simulink model "ZEM_Example"  (R2020b)
settings: Solver=ode4  StartTime=0.0  StopTime=simTime  FixedStep=h  RelTol=1e-3
values from neighbouring files (symbols this model uses):
  Beta = 0    [ZeroEffortMiss.m]
  N_prime = 4    [ZeroEffortMiss.m]
  nt = 3    [ZeroEffortMiss.m]
  Rm1 = 0    [ZeroEffortMiss.m]
  Rm2 = 10000    [ZeroEffortMiss.m]
  Rt1 = 40000    [ZeroEffortMiss.m]
  Rt2 = Rm2    (= 10000)    [ZeroEffortMiss.m]
  Tf = simTime    (= 10)    [ZeroEffortMiss.m]
  Vm1_0 = Vm*cos(L+HE+Lambda)    [ZeroEffortMiss.m]
  Vm2_0 = Vm*sin(L+HE+Lambda)    [ZeroEffortMiss.m]
  Vt = 1000    [ZeroEffortMiss.m]
  Vt1_0 = -Vt*cos(Beta)    [ZeroEffortMiss.m]
  Vt2_0 = Vt*sin(Beta)    [ZeroEffortMiss.m]
libraries: simulink x1
settings Model: Creator=dariusmensah  LastModifiedBy=dariusmensah

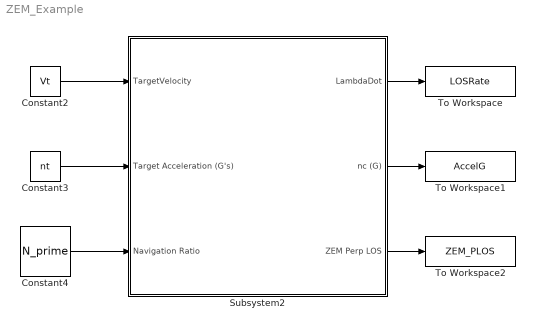
== system ZEM_Example ==
  Constant2 : Constant  Value=Vt
  Constant3 : Constant  Value=nt
  Constant4 : Constant  Value=N_prime
  Subsystem2 : Subsystem
  To Workspace : ToWorkspace  VariableName=LOSRate  SaveFormat=Structure With Time  SampleTime=-1
  To Workspace1 : ToWorkspace  VariableName=AccelG  SaveFormat=Structure With Time  SampleTime=-1
  To Workspace2 : ToWorkspace  VariableName=ZEM_PLOS  SaveFormat=Structure With Time  SampleTime=-1
  wires:
  Constant2/1 -> Subsystem2/1(TargetVelocity)
  Constant4/1 -> Subsystem2/3(Navigation Ratio)
  Constant3/1 -> Subsystem2/2(Target Acceleration (G's))
  Subsystem2/3(ZEM Perp LOS) -> To Workspace2/1
  Subsystem2/2(nc (G)) -> To Workspace1/1
  Subsystem2/1(LambdaDot) -> To Workspace/1

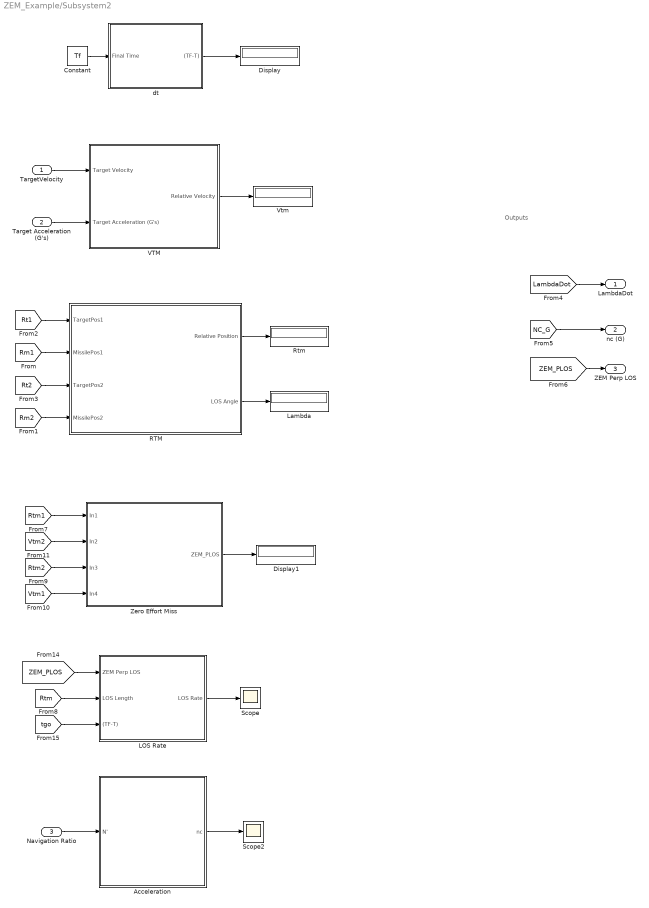
== system ZEM_Example/Subsystem2 ==
  note: Outputs
  TargetVelocity : Inport
  Target Acceleration (G's) : Inport  Port=2
  Navigation Ratio : Inport  Port=3
  Acceleration : Subsystem
  Constant : Constant  Value=Tf
  Display : Display
  Display1 : Display
  LOS Rate : Subsystem
  Lambda : Display
  RTM : Subsystem
  Rtm : Display
  Scope : Scope
  Scope2 : Scope
  VTM : Subsystem
  Vtm : Display
  Zero Effort Miss : Subsystem
  dt : Subsystem
  LambdaDot : Outport
  nc (G) : Outport  Port=2
  ZEM Perp LOS : Outport  Port=3
  wires:
  TargetVelocity/1 -> VTM/1(Target Velocity)
  [Rm2] -> RTM/4(MissilePos2)
  [Rt1] -> RTM/1(TargetPos1)
  VTM/1(Relative Velocity) -> Vtm/1
  RTM/1(Relative Position) -> Rtm/1
  [Rt2] -> RTM/3(TargetPos2)
  [Rm1] -> RTM/2(MissilePos1)
  Target Acceleration (G's)/1 -> VTM/2(Target Acceleration (G's))
  RTM/2(LOS Angle) -> Lambda/1
  Navigation Ratio/1 -> Acceleration/1(N')
  Acceleration/1(nc) -> Scope2/1
  [ZEM_PLOS] -> LOS Rate/1(ZEM Perp LOS)
  [Rtm] -> LOS Rate/2(LOS Length)
  [tgo] -> LOS Rate/3((TF-T))
  LOS Rate/1(LOS Rate) -> Scope/1
  Constant/1 -> dt/1(Final Time)
  dt/1((TF-T)) -> Display/1
  Zero Effort Miss/1(ZEM_PLOS) -> Display1/1
  [LambdaDot] -> LambdaDot/1
  [NC_G] -> nc (G)/1
  [ZEM_PLOS] -> ZEM Perp LOS/1
  [Rtm1] -> Zero Effort Miss/1(In1)
  [Vtm2] -> Zero Effort Miss/2(In2)
  [Rtm2] -> Zero Effort Miss/3(In3)
  [Vtm1] -> Zero Effort Miss/4(In4)

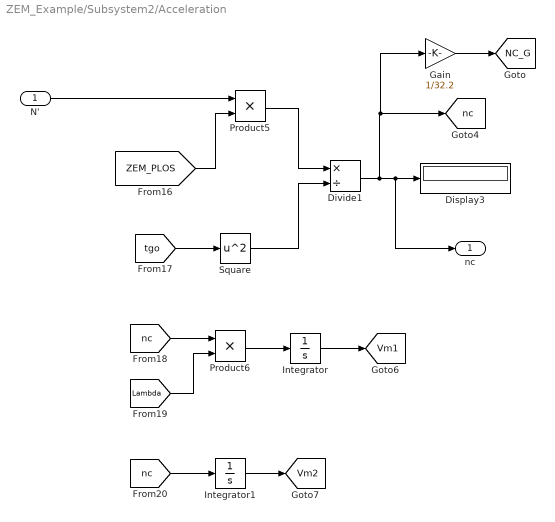
== system ZEM_Example/Subsystem2/Acceleration ==
  N' : Inport
  Display3 : Display
  Divide1 : Product  Inputs=*/
  Gain : Gain  Gain=1/32.2
  Integrator : Integrator  InitialCondition=Vm1_0
  Integrator1 : Integrator  InitialCondition=Vm2_0
  Product5 : Product
  Product6 : Product
  Square : Math  Operator=square  SaturateOnIntegerOverflow=on
  nc : Outport
  tag scope: NC_G=global, Vm1=global, Vm2=global, nc=global
  wires:
  [nc] -> Product6/1
  [tgo] -> Square/1
  N'/1 -> Product5/1
  Integrator1/1 -> [Vm2]
  [Lambda] -> Product6/2
  Integrator/1 -> [Vm1]
  Square/1 -> Divide1/2
  Product5/1 -> Divide1/1
  [ZEM_PLOS] -> Product5/2
  Divide1/1 -> Gain/1, [nc], nc/1, Display3/1
  Product6/1 -> Integrator/1
  Gain/1 -> [NC_G]
  [nc] -> Integrator1/1

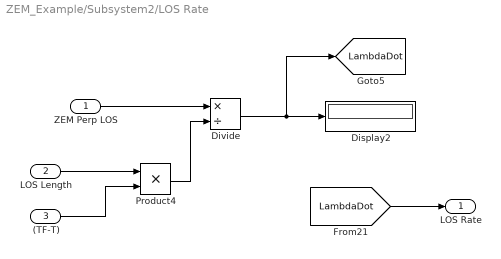
== system ZEM_Example/Subsystem2/LOS Rate ==
  ZEM Perp LOS : Inport
  LOS Length : Inport  Port=2
  (TF-T) : Inport  Port=3
  Display2 : Display
  Divide : Product  Inputs=*/
  Product4 : Product
  LOS Rate : Outport
  tag scope: LambdaDot=global
  wires:
  (TF-T)/1 -> Product4/2
  LOS Length/1 -> Product4/1
  Divide/1 -> [LambdaDot], Display2/1
  [LambdaDot] -> LOS Rate/1
  Product4/1 -> Divide/2
  ZEM Perp LOS/1 -> Divide/1

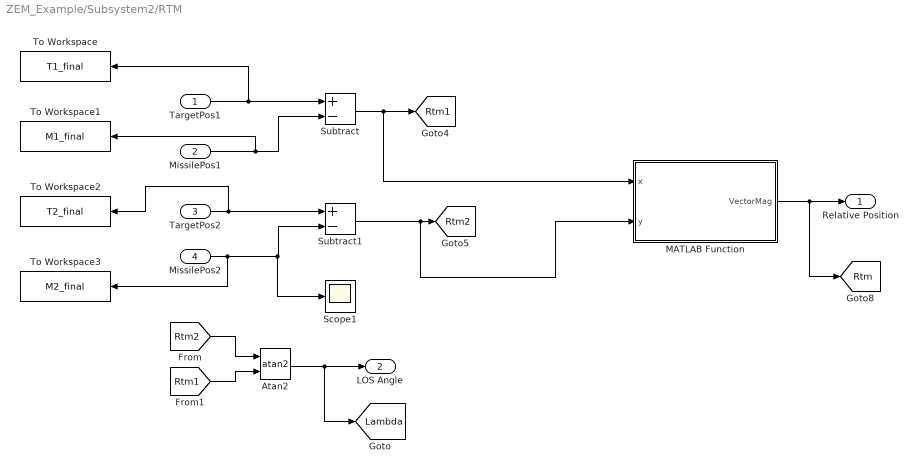
== system ZEM_Example/Subsystem2/RTM ==
  TargetPos1 : Inport
  MissilePos1 : Inport  Port=2
  TargetPos2 : Inport  Port=3
  MissilePos2 : Inport  Port=4
  Atan2 : Trigonometry  Operator=atan2
  MATLAB Function : MATLAB Function  TreatAsAtomicUnit=on
  Scope1 : Scope
  Subtract : Sum  Inputs=+-
  Subtract1 : Sum  Inputs=+-
  To Workspace : ToWorkspace  VariableName=T1_final  SaveFormat=Structure With Time  SampleTime=-1
  To Workspace1 : ToWorkspace  VariableName=M1_final  SaveFormat=Structure With Time  SampleTime=-1
  To Workspace2 : ToWorkspace  VariableName=T2_final  SaveFormat=Structure With Time  SampleTime=-1
  To Workspace3 : ToWorkspace  VariableName=M2_final  SaveFormat=Structure With Time  SampleTime=-1
  Relative Position : Outport
  LOS Angle : Outport  Port=2
  tag scope: Lambda=global, Rtm1=global, Rtm2=global, Rtm=global
  wires:
  MissilePos2/1 -> To Workspace3/1, Scope1/1, Subtract1/2
  Subtract1/1 -> MATLAB Function/2(y), [Rtm2]
  TargetPos1/1 -> To Workspace/1, Subtract/1
  TargetPos2/1 -> To Workspace2/1, Subtract1/1
  Subtract/1 -> MATLAB Function/1(x), [Rtm1]
  MissilePos1/1 -> To Workspace1/1, Subtract/2
  [Rtm1] -> Atan2/2
  [Rtm2] -> Atan2/1
  Atan2/1 -> [Lambda], LOS Angle/1
  MATLAB Function/1(VectorMag) -> [Rtm], Relative Position/1

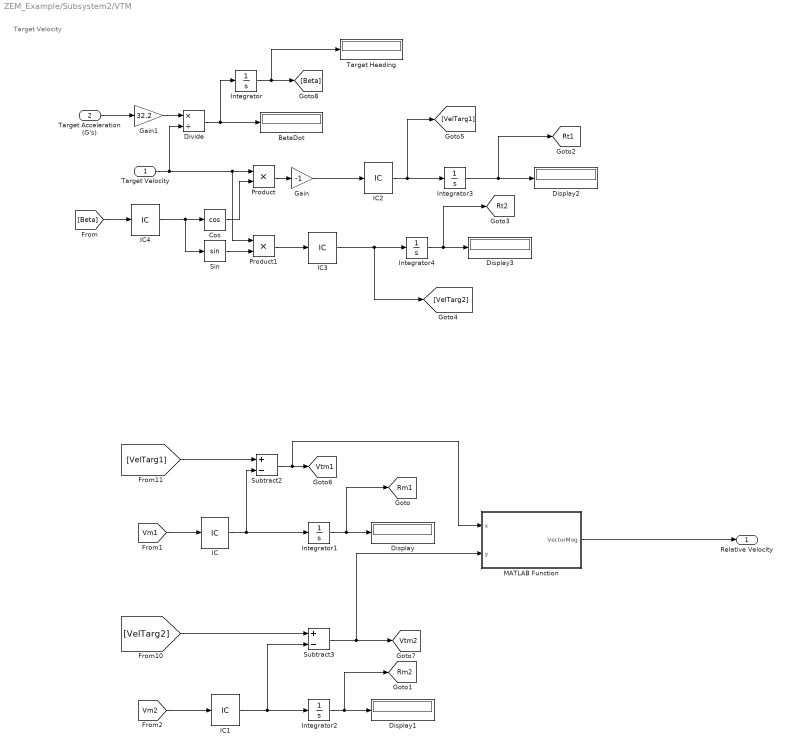
== system ZEM_Example/Subsystem2/VTM ==
  note: Target Velocity
  Target Velocity : Inport
  Target Acceleration (G's) : Inport  Port=2
  BetaDot : Display
  Cos : Trigonometry  Operator=cos
  Display{,1..3} (4 alike) : Display
  Divide : Product  Inputs=*/
  Gain : Gain  Gain=-1
  Gain1 : Gain  Gain=32.2
  IC : InitialCondition  Value=Vm1_0
  IC1 : InitialCondition  Value=Vm2_0
  IC2 : InitialCondition  Value=Vt1_0
  IC3 : InitialCondition  Value=Vt2_0
  IC4 : InitialCondition  Value=Beta
  Integrator : Integrator
  Integrator1 : Integrator  InitialCondition=Rm1
  Integrator2 : Integrator  InitialCondition=Rm2
  Integrator3 : Integrator  InitialCondition=Rt1
  Integrator4 : Integrator  InitialCondition=Rt2
  MATLAB Function : MATLAB Function  TreatAsAtomicUnit=on
  Product : Product
  Product1 : Product
  Sin : Trigonometry
  Subtract2 : Sum  Inputs=+-
  Subtract3 : Sum  Inputs=+-
  Target Heading : Display
  Relative Velocity : Outport
  tag scope: Rm1=global, Rm2=global, Rt1=global, Rt2=global, Vtm1=global, Vtm2=global
  wires:
  MATLAB Function/1(VectorMag) -> Relative Velocity/1
  [Vm1] -> IC/1
  Sin/1 -> Product1/2
  [VelTarg1] -> Subtract2/1
  Product/1 -> Gain/1
  Target Velocity/1 -> Divide/2, Product1/1, Product/1
  Subtract2/1 -> MATLAB Function/1(x), [Vtm1]
  [VelTarg2] -> Subtract3/1
  Cos/1 -> Product/2
  Product1/1 -> IC3/1
  Subtract3/1 -> MATLAB Function/2(y), [Vtm2]
  Integrator4/1 -> [Rt2], Display3/1
  IC/1 -> Integrator1/1, Subtract2/2
  [Vm2] -> IC1/1
  [Beta] -> IC4/1
  IC2/1 -> [VelTarg1], Integrator3/1
  Integrator2/1 -> [Rm2], Display1/1
  IC3/1 -> [VelTarg2], Integrator4/1
  Integrator1/1 -> Display/1, [Rm1]
  Integrator3/1 -> Display2/1, [Rt1]
  IC1/1 -> Subtract3/2, Integrator2/1
  Gain/1 -> IC2/1
  Divide/1 -> BetaDot/1, Integrator/1
  IC4/1 -> Sin/1, Cos/1
  Integrator/1 -> Target Heading/1, [Beta]
  Target Acceleration (G's)/1 -> Gain1/1
  Gain1/1 -> Divide/1

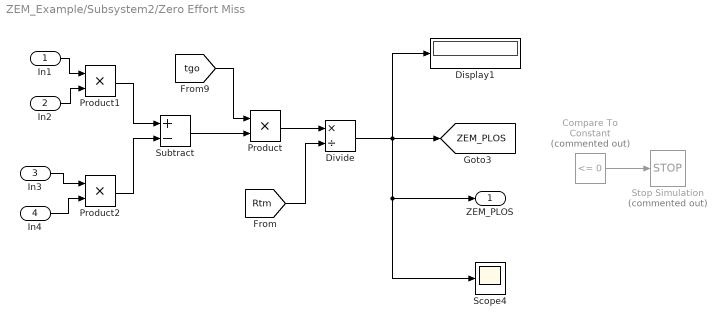
== system ZEM_Example/Subsystem2/Zero Effort Miss ==
  In1 : Inport
  In2 : Inport  Port=2
  In3 : Inport  Port=3
  In4 : Inport  Port=4
  Compare To Constant : simulink/Logic and Bit Operations/Compare To Constant  Commented=on  relop=<=  const=0  OutDataTypeStr=boolean
  Display1 : Display
  Divide : Product  Inputs=*/
  Product : Product
  Product1 : Product
  Product2 : Product
  Scope4 : Scope
  Stop Simulation : Stop  Commented=on
  Subtract : Sum  Inputs=+-
  ZEM_PLOS : Outport
  tag scope: ZEM_PLOS=global
  wires:
  Compare To Constant/1 -> Stop Simulation/1
  In2/1 -> Product1/2
  In1/1 -> Product1/1
  Product1/1 -> Subtract/1
  In3/1 -> Product2/1
  In4/1 -> Product2/2
  Product2/1 -> Subtract/2
  Subtract/1 -> Product/2
  [tgo] -> Product/1
  Product/1 -> Divide/1
  [Rtm] -> Divide/2
  Divide/1 -> Display1/1, Scope4/1, ZEM_PLOS/1, [ZEM_PLOS]

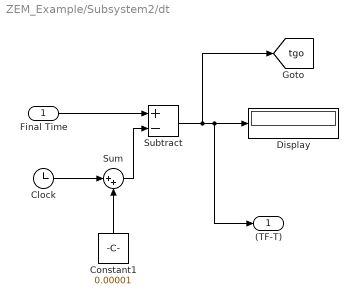
== system ZEM_Example/Subsystem2/dt ==
  Final Time : Inport
  Clock : Clock
  Constant1 : Constant  Value=0.00001
  Display : Display
  Subtract : Sum  Inputs=+-
  Sum : Sum  Inputs=|++
  (TF-T) : Outport
  tag scope: tgo=global
  wires:
  Final Time/1 -> Subtract/1
  Sum/1 -> Subtract/2
  Clock/1 -> Sum/1
  Subtract/1 -> [tgo], (TF-T)/1, Display/1
  Constant1/1 -> Sum/2

== matlab function ZEM_Example/Subsystem2/RTM/MATLAB Function ==
  data: x input; VectorMag output; y input
function VectorMag = fcn(x,y)

a = x^2 + y^2;
VectorMag = sqrt(a);
end

== matlab function ZEM_Example/Subsystem2/VTM/MATLAB Function ==
  data: x input; VectorMag output; y input
function VectorMag = fcn(x,y)

a = x^2 + y^2;
VectorMag = sqrt(a);
end
